simulink model "HSX_test2_0214"  (R2023b)
settings: Solver=VariableStepAuto  StartTime=0.0  StopTime=40  RelTol=1e-3
values from neighbouring files (symbols this model uses):
  Iref1 = 8600    [Start.m]
  LHSX = 0.02    [Start.m]    (also in Verification.m; cehck.m)
  Ra = 0.0096    [Start.m]    (also in Verification.m; cehck.m)
  RHSX = 0.09    [Start.m]    (also in Verification.m; cehck.m)
  Vf = 0.6    [Start.m]    (also in Verification.m = 4.5; cehck.m = 3.1)
libraries: spsIdealSwitchLib x2, spsVoltageMeasurementLib x2, spsSeriesRLCBranchLib x1, spsControlledVoltageSourceLib x1, spsCurrentMeasurementLib x1, spsDCMachineLib x1, spsDiodeLib x1, sps_lib x1
settings Model: Creator=Hyeongmeen  LastModifiedBy=Hyeongmeen

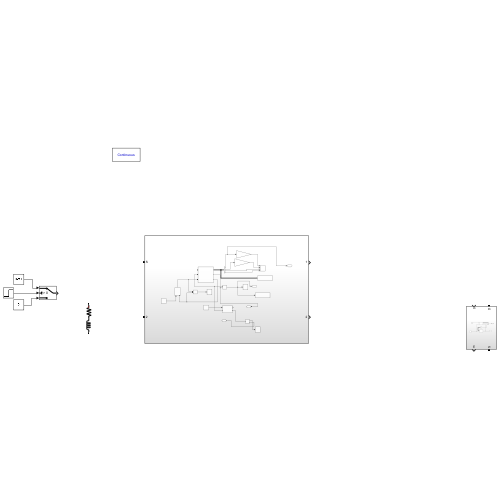
[thumbnail: Simulink's stored preview of the top-level diagram]
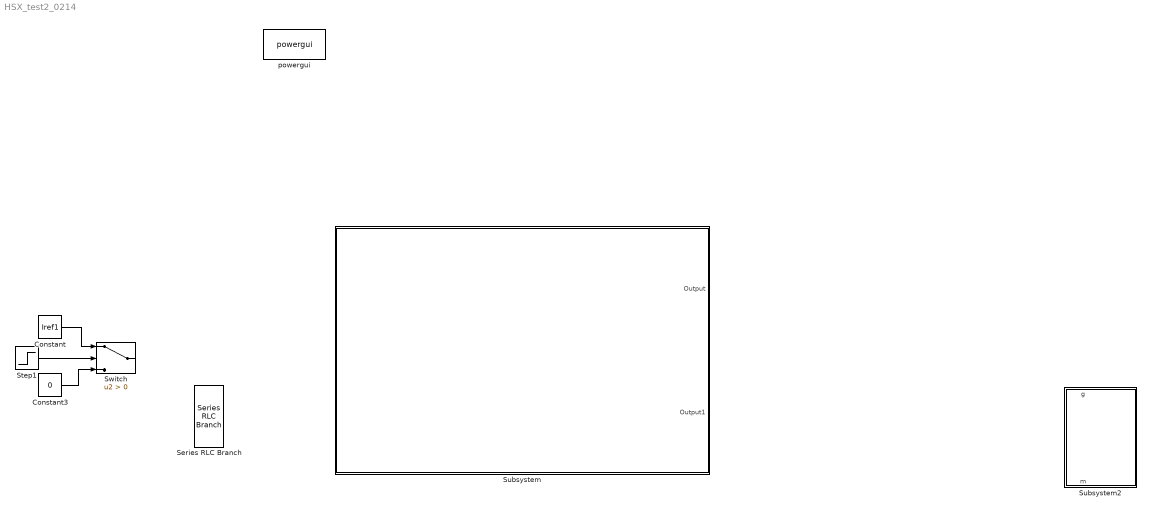
== system HSX_test2_0214 ==
  Constant : Constant  Value=Iref1
  Constant3 : Constant  Value=0
  Series RLC Branch : spsSeriesRLCBranchLib/Series RLC Branch  LConnTagsString=__new0  RConnTagsString=__new0  BranchType=RL  Resistance=RHSX  Inductance=16*LHSX  SetiL0=off  InitialCurrent=0  Capacitance=1e-6  Setx0=off  InitialVoltage=0  Measurements=None
  Step1 : Step  Time=21  SampleTime=0  VectorParams1D=off  ZeroCross=off
  Subsystem : Subsystem
  Subsystem2 : Subsystem
  Switch : Switch  Criteria=u2 > Threshold  SaturateOnIntegerOverflow=off  InputSameDT=off
  powergui : sps_lib/powergui  Priority=1  SimulationMode=Continuous  SampleTime=1e-7  frequency=60  Iterations=50  frequencyindice=0  Pbase=100e6  ErrMax=1e-4  UnitsV=kV  UnitsW=MW  buscounter=0  FunctionMessages=off  echomessages=off  EnableUseOfTLC=off  CurrentSourceSwitches=off  DisableSnubberDevices=off  DisableRonSwitches=off  DisableVfSwitches=off  DisplayEquations=off  AutomaticDiscreteSolvers=off  SolverType=Tustin/Backward Euler (TBE)  Interpol=off  ExternalGateDelay=off  methode=off  Ts=100  x0status=blocks  SPID=on  SwTol=0  HookPort=off  NonlinearTolerance=1e-4  nMaxIteration=100  ContinueOnMaxIteration=off  RestoreLinks=warning  ResistiveCurrentMeasurement=off  Frange=[0:2:500]  Ylog=off  Xlog=on  ShowGrid=off  save=off  variable=ZData  structure=0  ZoomFFT=off  StartTime=0.0  cycles=1  DisplayStyle=1  fundamental=60  FreqAxis=off  MaxFrequency=1000  frequencyindicesteady=1  RmsSteady=1  display=off
  wires:
  Constant3/1 -> Switch/3
  Step1/1 -> Switch/2
  Constant/1 -> Switch/1

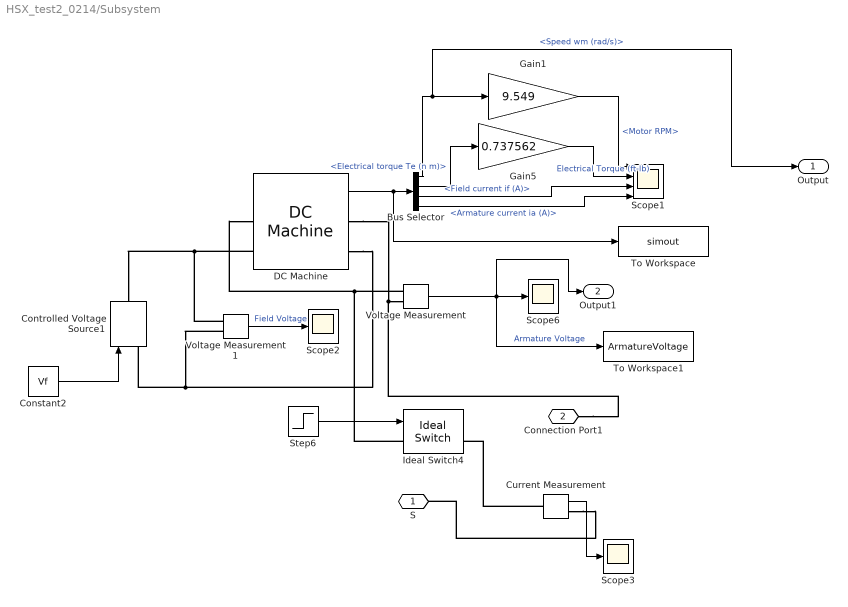
== system HSX_test2_0214/Subsystem ==
  Bus Selector : BusSelector  OutputSignals=Speed wm (rad/s),Electrical torque Te (n m),Field current if (A),Armature current ia (A)
  Constant2 : Constant  Value=Vf
  Controlled Voltage Source1 : spsControlledVoltageSourceLib/Controlled Voltage Source  Initialize=on  Source_Type=DC  Amplitude=0  Phase=0  Frequency=0  Measurements=Voltage
  Current Measurement : spsCurrentMeasurementLib/Current Measurement  PhasorSimulation=off  OutputType=Complex  PSBequivalent=0
  DC Machine : spsDCMachineLib/DC Machine  PresetModel=No  MechanicalLoad=Torque TL  FieldType=Wound  ShowDetailedParameters=on  MeasurementBus=off  RLa="[Ra  0.002]"  RLf=[0.0054 0.0125]  Laf=Laf  MachineConstant=Torque constant (N.m/A)  Ke=1.8  Kt=1.8  J=137  Bm=0  Tf=0  w0=w_initial  Ifinit=0  TsPowergui=0  TsBlock=-1
  Gain1 : Gain  Gain=9.549
  Gain5 : Gain  Gain=0.737562
  Ideal Switch4 : spsIdealSwitchLib/Ideal Switch  Ron=0  Lon=0  IC=0  Rs=inf  Cs=0  Measurements=on
  Scope1 : Scope  NumInputPorts=4
  Scope2 : Scope
  Scope3 : Scope
  Scope6 : Scope
  Step6 : Step  Time=20  SampleTime=0  VectorParams1D=off  ZeroCross=off
  To Workspace : ToWorkspace  VariableName=simout  SaveFormat=Timeseries  SampleTime=-1
  To Workspace1 : ToWorkspace  VariableName=ArmatureVoltage  SaveFormat=Timeseries  SampleTime=-1
  Voltage Measurement : spsVoltageMeasurementLib/Voltage Measurement  PhasorSimulation=off  OutputType=Complex  PSBequivalent=0
  Voltage Measurement1 : spsVoltageMeasurementLib/Voltage Measurement  PhasorSimulation=off  OutputType=Complex  PSBequivalent=0
  S : PMIOPort  Side=Left
  Connection Port1 : PMIOPort  Port=2  Side=Left
  Output : Outport
  Output1 : Outport  Port=2
  wires:
  Voltage Measurement/1 -> To Workspace1/1, Scope6/1, Output1/1  "Armature Voltage"
  Voltage Measurement1/1 -> Scope2/1  "Field Voltage"
  Constant2/1 -> Controlled Voltage Source1/1
  Current Measurement/1 -> Scope3/1
  DC Machine/1 -> To Workspace/1, Bus Selector/1
  Gain1/1 -> Scope1/1  "<Motor RPM>"
  Bus Selector/3 -> Scope1/3  "<Field current if (A)>"
  Bus Selector/2 -> Gain5/1  "<Electrical torque Te (n m)>"
  Bus Selector/4 -> Scope1/4  "<Armature current ia (A)>"
  Bus Selector/1 -> Output/1, Gain1/1  "<Speed wm (rad/s)>"
  Gain5/1 -> Scope1/2  "Electrical Torque (ft-lb)"
  Step6/1 -> Ideal Switch4/1
  connections:
  DC Machine/RConn1 -- Connection Port1/RConn1 -- Voltage Measurement/LConn2
  Voltage Measurement/LConn1 -- Ideal Switch4/LConn1 -- DC Machine/LConn1
  DC Machine/LConn2 -- Voltage Measurement1/LConn1 -- Controlled Voltage Source1/RConn1
  DC Machine/RConn2 -- Voltage Measurement1/LConn2 -- Controlled Voltage Source1/LConn1
  Current Measurement/LConn1 -- Ideal Switch4/RConn1
  Current Measurement/RConn1 -- S/RConn1

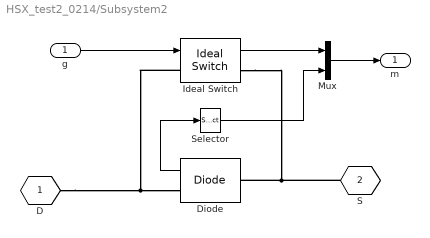
== system HSX_test2_0214/Subsystem2 ==
  g : Inport
  Diode : spsDiodeLib/Diode  Ron=1e-3  Lon=0  Vf=Vf  IC=0  UseSnubber=0  Rs=inf  Cs=0  Measurements=on
  Ideal Switch : spsIdealSwitchLib/Ideal Switch  Ron=1e-3  Lon=0  IC=0  Rs=Rs_fet  Cs=Cs_fet  Measurements=on
  Mux : Mux  Inputs=[2,1]
  Selector : Selector  InputPortWidth=2  IndexOptions=Index vector (dialog)  Indices=1  OutputSizes=1
  D : PMIOPort  Tag=PMCPort  Side=Left
  S : PMIOPort  Tag=PMCPort  Port=2  Side=Right
  m : Outport  VectorParamsAs1DForOutWhenUnconnected=off
  wires:
  Ideal Switch/1 -> Mux/1
  Diode/1 -> Selector/1
  Mux/1 -> m/1
  g/1 -> Ideal Switch/1
  Selector/1 -> Mux/2
  connections:
  Ideal Switch/LConn1 -- Diode/RConn1 -- D/RConn1
  Ideal Switch/RConn1 -- Diode/LConn1 -- S/RConn1
